simulink model "scheduling_integral_contoller_with_observer"  (R2016a)
settings: Solver=VariableStepAuto  StartTime=0.0  StopTime=.10  RelTol=1e-5
undefined symbols (not defined in the file or in its folder): A, A_lt, B, B_lt, C, C_lt, K, Ki_lt, Ko, Ko_lt, ws_lt
settings Model: Creator=manuel  LastModifiedBy=manuel

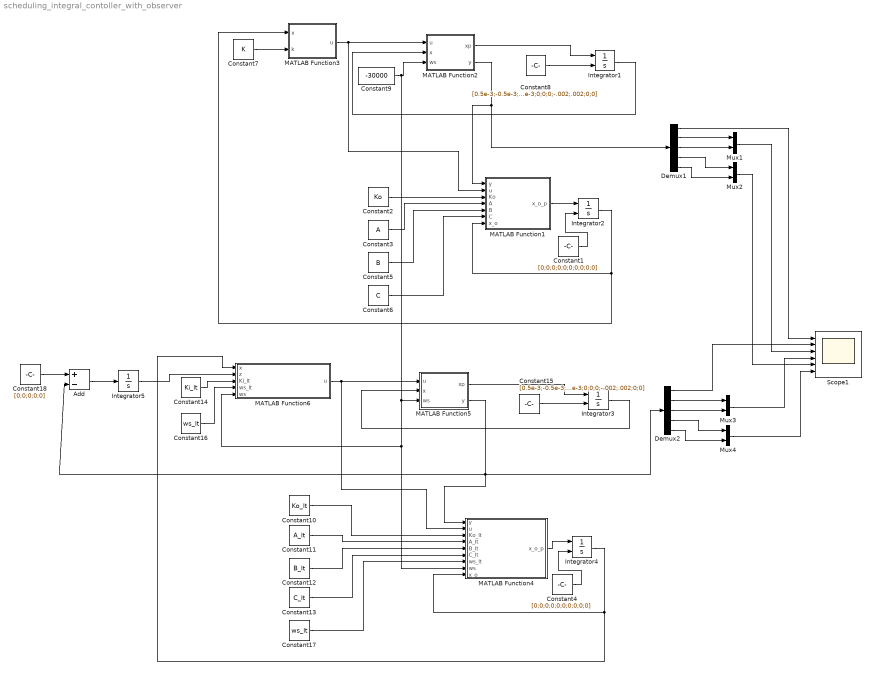
== system scheduling_integral_contoller_with_observer ==
  Add : Sum  Inputs=+-
  Constant1 : Constant  Value=[0;0;0;0;0;0;0;0;0;0]
  Constant10 : Constant  Value=Ko_lt  VectorParams1D=off
  Constant11 : Constant  Value=A_lt  VectorParams1D=off
  Constant12 : Constant  Value=B_lt  VectorParams1D=off
  Constant13 : Constant  Value=C_lt  VectorParams1D=off
  Constant14 : Constant  Value=Ki_lt  VectorParams1D=off
  Constant15 : Constant  Value=[0.5e-3;-0.5e-3;1e-3;0;0;0;-.002;.002;0;0]
  Constant16 : Constant  Value=ws_lt  VectorParams1D=off
  Constant17 : Constant  Value=ws_lt  VectorParams1D=off
  Constant18 : Constant  Value=[0;0;0;0;0]
  Constant2 : Constant  Value=Ko  VectorParams1D=off
  Constant3 : Constant  Value=A  VectorParams1D=off
  Constant4 : Constant  Value=[0;0;0;0;0;0;0;0;0;0]
  Constant5 : Constant  Value=B  VectorParams1D=off
  Constant6 : Constant  Value=C  VectorParams1D=off
  Constant7 : Constant  Value=K  VectorParams1D=off
  Constant8 : Constant  Value=[0.5e-3;-0.5e-3;1e-3;0;0;0;-.002;.002;0;0]
  Constant9 : Constant  Value=-30000  VectorParams1D=off
  Demux1 : Demux  Outputs=5
  Demux2 : Demux  Outputs=5
  Integrator{1..4} (4 alike) : Integrator  InitialConditionSource=external
  Integrator5 : Integrator  InitialCondition=[0;0;0;0;0]
  MATLAB Function1 : MATLAB Function  TreatAsAtomicUnit=on
  MATLAB Function2 : MATLAB Function  TreatAsAtomicUnit=on
  MATLAB Function3 : MATLAB Function  TreatAsAtomicUnit=on
  MATLAB Function4 : MATLAB Function  TreatAsAtomicUnit=on
  MATLAB Function5 : MATLAB Function  TreatAsAtomicUnit=on
  MATLAB Function6 : MATLAB Function  TreatAsAtomicUnit=on
  Mux{1..4} (4 alike) : Mux  Inputs=2
  Scope1 : Scope  NumInputPorts=6
  wires:
  Constant8/1 -> Integrator1/2
  Integrator1/1 -> MATLAB Function2/2(x)
  Constant7/1 -> MATLAB Function3/2(k)
  MATLAB Function2/1(xp) -> Integrator1/1
  MATLAB Function2/2(y) -> Demux1/1, MATLAB Function1/1(y)
  Constant1/1 -> Integrator2/2
  MATLAB Function1/1(x_o_p) -> Integrator2/1
  Constant2/1 -> MATLAB Function1/3(Ko)
  Constant3/1 -> MATLAB Function1/4(A)
  Constant5/1 -> MATLAB Function1/5(B)
  Constant6/1 -> MATLAB Function1/6(C)
  Integrator2/1 -> MATLAB Function3/1(x), MATLAB Function1/7(x_o)
  MATLAB Function3/1(u) -> MATLAB Function1/2(u), MATLAB Function2/1(u)
  Constant15/1 -> Integrator3/2
  Integrator3/1 -> MATLAB Function5/2(x)
  Constant14/1 -> MATLAB Function6/3(Ki_lt)
  MATLAB Function5/1(xp) -> Integrator3/1
  Constant4/1 -> Integrator4/2
  MATLAB Function4/1(x_o_p) -> Integrator4/1
  Constant10/1 -> MATLAB Function4/3(Ko_lt)
  Constant11/1 -> MATLAB Function4/4(A_lt)
  Constant12/1 -> MATLAB Function4/5(B_lt)
  Constant13/1 -> MATLAB Function4/6(C_lt)
  Integrator4/1 -> MATLAB Function4/9(x_o), MATLAB Function6/1(x)
  MATLAB Function6/1(u) -> MATLAB Function4/2(u), MATLAB Function5/1(u)
  Constant9/1 -> MATLAB Function6/5(ws), MATLAB Function4/8(ws), MATLAB Function5/3(ws), MATLAB Function2/3(ws)
  Constant16/1 -> MATLAB Function6/4(ws_lt)
  Constant17/1 -> MATLAB Function4/7(ws_lt)
  Demux1/1 -> Scope1/1
  Demux1/2 -> Mux1/1
  Demux1/3 -> Mux1/2
  Mux1/1 -> Scope1/3
  Mux2/1 -> Scope1/5
  Demux1/4 -> Mux2/1
  Demux1/5 -> Mux2/2
  Demux2/2 -> Mux3/1
  Demux2/3 -> Mux3/2
  Demux2/4 -> Mux4/1
  Demux2/5 -> Mux4/2
  MATLAB Function5/2(y) -> Add/2, MATLAB Function4/1(y), Demux2/1
  Mux3/1 -> Scope1/4
  Mux4/1 -> Scope1/6
  Demux2/1 -> Scope1/2
  Add/1 -> Integrator5/1
  Constant18/1 -> Add/1
  Integrator5/1 -> MATLAB Function6/2(z)

== matlab function scheduling_integral_contoller_with_observer/MATLAB Function1 ==
  data: y input; u input; x_o_p output; Ko input; A input; B input; C input; x_o input
function x_o_p = state_obsever(y,u,Ko,A,B,C,x_o)
%#codegen
x_o_p = A*x_o + B*u + Ko*(y-C*x_o);

== matlab function scheduling_integral_contoller_with_observer/MATLAB Function4 ==
  data: y input; u input; x_o_p output; Ko_lt input; A_lt input; B_lt input; C_lt input; ws_lt input; ws input; x_o input
function x_o_p = state_obsever(y,u,Ko_lt,A_lt,B_lt,C_lt,ws_lt,ws,x_o)
%#codegen
Ko = matrix_interpolation(ws_lt,Ko_lt,ws);
A = matrix_interpolation(ws_lt,A_lt,ws);
B = matrix_interpolation(ws_lt,B_lt,ws);
C = matrix_interpolation(ws_lt,C_lt,ws);

x_o_p = A*x_o + B*u + Ko*(y-C*x_o);

== matlab function scheduling_integral_contoller_with_observer/MATLAB Function2 ==
  data: u input; x input; xp output; y output; ws input
function [xp,y] = fcn(u,x,ws)

Fd_x = 0;
Fd_y = 0;
Fd_z = 0;
Md_y = 0;
Md_z = 0;
[xp,y] = hmb_non_linear_model(x,u,ws,Fd_x,Fd_y,Fd_z,Md_y,Md_z);

end

== matlab function scheduling_integral_contoller_with_observer/MATLAB Function3 ==
  data: x input; k input; u output
function u = feedback_controller(x,k)
%#codegen
u = -k*x;

== matlab function scheduling_integral_contoller_with_observer/MATLAB Function5 ==
  data: u input; x input; xp output; y output; ws input
function [xp,y] = fcn(u,x,ws)

Fd_x = 0;
Fd_y = 0;
Fd_z = 0;
Md_y = 0;
Md_z = 0;
[xp,y] = hmb_non_linear_model(x,u,ws,Fd_x,Fd_y,Fd_z,Md_y,Md_z);

end

== matlab function scheduling_integral_contoller_with_observer/MATLAB Function6 ==
  data: x input; z input; Ki_lt input; ws_lt input; u output; ws input
function u  = feedback_controller(x,z,Ki_lt,ws_lt,ws)
%#codegen
ki = matrix_interpolation(ws_lt,Ki_lt,ws);

xi = [x;z];

u = -ki*xi;
